simulink model "matlabFcnExample"  (R2015a)
settings: Solver=ode45  StartTime=0.0  StopTime=10.0  RelTol=1e-3
undefined symbols (not defined in the file or in its folder): A
settings Model: Creator=John  LastModifiedBy=John

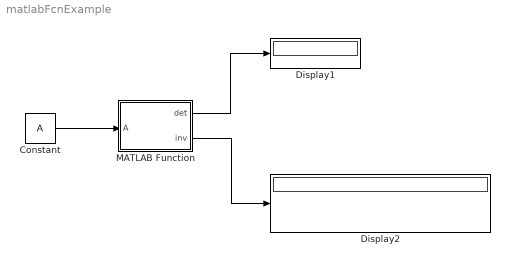
== system matlabFcnExample ==
  Constant : Constant  Value=A
  Display1 : Display
  "Display2 " : Display
  MATLAB Function : MATLAB Function  TreatAsAtomicUnit=on
  wires:
  MATLAB Function/1(det) -> Display1/1
  Constant/1 -> MATLAB Function/1(A)
  MATLAB Function/2(inv) -> "Display2 "/1

== matlab function matlabFcnExample/MATLAB Function ==
  data: A input; det output; inv output
function [det, inv] = matrix(A)
% This function computes the determinant and the inverse of a 3x3
% matrix A which must be defined in MATLAB's Command Window.
%

det=A(1,1)*A(2,2)*A(3,3)+A(1,2)*A(2,3)*A(3,1)+A(1,3)*A(2,1)*A(3,2)...
-A(3,1)*A(2,2)*A(1,3)-A(3,2)*A(2,3)*A(1,1)-A(3,3)*A(2,1)*A(1,2);
%
% For a 3x3 matrix where A=[a11 a12 a13; a21 a22 a23; a31 a32 a33],
% the inverse of A is obtained as invA = (1/detA)*adjA where adjA
% represents the adjoint of A. Ref: Numerical Analysis, ISBN 0-9709511-1-6
% The cofactors are defined below.
%
b11 = A(2,2)*A(3,3)-A(2,3)*A(3,2);
b12 = -(A(2,1)*A(3,3)-A(2,3)*A(3,1));
b13 = A(2,1)*A(3,2)-A(2,2)*A(3,1);
b21 = -(A(1,2)*A(3,3)-A(1,3)*A(3,2));
b22 = A(1,1)*A(3,3)-A(1,3)*A(3,1);
b23 = -(A(1,1)*A(3,2)-A(1,2)*A(3,1));
b31 = A(1,2)*A(2,3)-A(1,3)*A(2,2);
b32 = -(A(1,1)*A(2,3)-A(1,3)*A(2,1));
b33 = A(1,1)*A(2,2)-A(1,2)*A(2,1);
% We must remember that the cofactors of the elemements of the ith
% row (column) of A are the elements of the ith column (row) of AdjA.
adjA = [b11 b12 b13; b21 b22 b23; b31 b32 b33]';
inv = (1/det)*adjA;
